simulink model "vehicle_body_v2"  (R2020b)
settings: Solver=VariableStepAuto  StartTime=0.0  StopTime=10.0  RelTol=1e-3
libraries: sdl_lib x14, nesl_utility x8, autolibshared x1
settings Model: Creator=True  LastModifiedBy=True

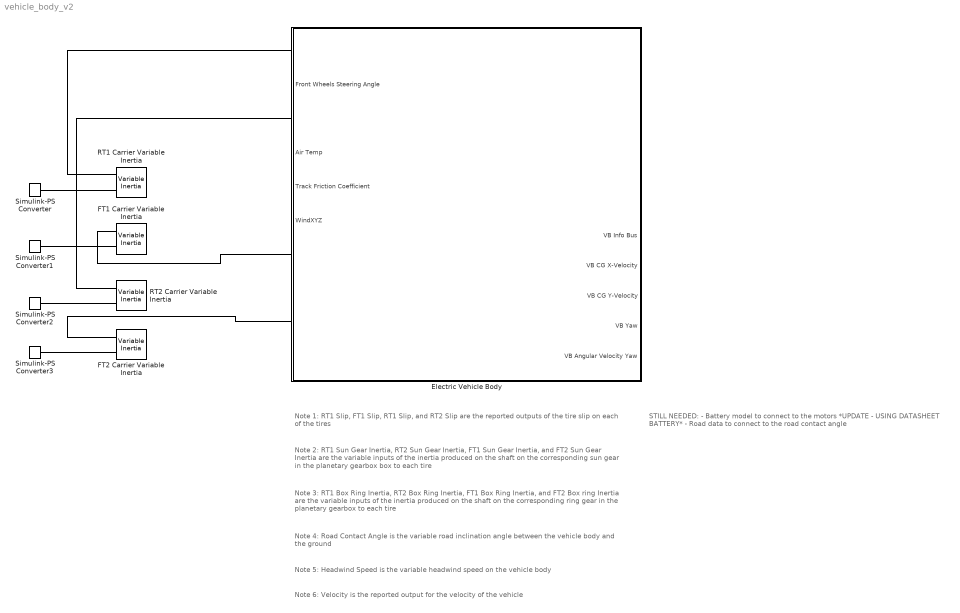
== system vehicle_body_v2 ==
  note: STILL NEEDED:
      |
      | - Battery model to connect to the motors *UPDATE - USING DATASHEET BATTERY*
      |
      | - Road data to connect to the road contact angle
  note: Note 6: Velocity is the reported output for the velocity of the vehicle
  note: Note 5: Headwind Speed is the variable headwind speed on the vehicle body
  note: Note 4: Road Contact Angle is the variable road inclination angle between the vehicle body and the ground
  note: Note 3: RT1 Box Ring Inertia, RT2 Box Ring Inertia, FT1 Box Ring Inertia, and FT2 Box ring Inertia are the variable inputs of the inertia produced on the shaft on the corresponding ring gear in the planetary gearbox to each tire
  note: Note 2: RT1 Sun Gear Inertia, RT2 Sun Gear Inertia, FT1 Sun Gear Inertia, and FT2 Sun Gear Inertia are the variable inputs of the inertia produced on the shaft on the corresponding sun gear in the planetary gearbox box to each tire
  note: Note 1: RT1 Slip, FT1 Slip, RT1 Slip, and RT2 Slip are the reported outputs of the tire slip on each of the tires
  Electric Vehicle Body : Subsystem
      settings: PortSchema="{\"entries\":[{\"content\":{\"sides\":[{\"content\":{\"connectorIds\":[\"LConn1\",\"In1\",\"LConn2\",\"In2\",\"In3\",\"In4\",\"LConn3\",\"LConn4\",\"LConn5\",\"LConn6\"]},\"type\":\"ConnectorPlacement.EquallySpacedRectSide\",\"uuid\":\"3589ffd8-3282-449f-9f73-db5573b89272\"},{\"content\":{\"connectorIds\":[\"RConn1\",\"RConn2\",\"RConn3\",\"RConn4\",\"RConn5\",\"RConn6\",\"Out1\",\"Out2\",\"Out3\",\"Out4\",\"Out5\"],\"side\":\"RIGHT\"},\"type\":\"ConnectorPlacement.EquallySpacedRectSide\",\"uuid\":\"4bc75fc4-5a6d-4cdc-a1d8-7589f1bfd0e3\"},{\"content\":{\"connectorIds\":[],\"side\":\"TOP\"},\"type\":\"ConnectorPlacement.EquallySpacedRectSide\",\"uuid\":\"5582f31c-489d-4354-9c03-0beb1d144974\"},{\"content\":{\"connectorIds\":[],\"side\":\"HIDDEN\"},\"type\":\"ConnectorPlacement.EquallySpacedRectSide\",\"uuid\":\"95051cab-6025-4def-8e94-855365c64cfc\"}]},\"type\":\"ConnectorPlacement.EquallySpacedConnector\",\"uuid\":\"f0af1aeb-7bbe-491f-85c8-fb0f3026e409\"}],\"packageUris\":[\"http://schema.mathworks.com/mf0/Connector/R2020b\"],\"version\":\"1.0\"}"
  FT1 Carrier Variable Inertia : sdl_lib/Inertias & Loads/Variable Inertia  minimum_inertia=0.1 kg*m^2  L_specify=off  L_priority=High  L=0 m^2*kg/s  L_nominal_specify=off  L_nominal_unit=m^2*kg/s  L_nominal_value=1
      settings: SourceProductBaseCode=LD  InternalSimscapePortConfiguration="{\"Bottom\":[],\"Left\":[{\"id\":\"I\",\"label\":\"\",\"type\":\"input\"},{\"id\":\"A\",\"label\":\"\",\"type\":\"foundation.mechanical.rotational.rotational\"}],\"Right\":[],\"Top\":[]}"
  FT2 Carrier Variable Inertia : sdl_lib/Inertias & Loads/Variable Inertia  minimum_inertia=0.1 kg*m^2  L_specify=off  L_priority=High  L=0 m^2*kg/s  L_nominal_specify=off  L_nominal_unit=m^2*kg/s  L_nominal_value=1
      settings: SourceProductBaseCode=LD  InternalSimscapePortConfiguration="{\"Bottom\":[],\"Left\":[{\"id\":\"I\",\"label\":\"\",\"type\":\"input\"},{\"id\":\"A\",\"label\":\"\",\"type\":\"foundation.mechanical.rotational.rotational\"}],\"Right\":[],\"Top\":[]}"
  RT1 Carrier Variable Inertia : sdl_lib/Inertias & Loads/Variable Inertia  minimum_inertia=0.1 kg*m^2  L_specify=off  L_priority=High  L=0 m^2*kg/s  L_nominal_specify=off  L_nominal_unit=m^2*kg/s  L_nominal_value=1
      settings: SourceProductBaseCode=LD  InternalSimscapePortConfiguration="{\"Bottom\":[],\"Left\":[{\"id\":\"I\",\"label\":\"\",\"type\":\"input\"},{\"id\":\"A\",\"label\":\"\",\"type\":\"foundation.mechanical.rotational.rotational\"}],\"Right\":[],\"Top\":[]}"
  RT2 Carrier Variable Inertia : sdl_lib/Inertias & Loads/Variable Inertia  minimum_inertia=0.1 kg*m^2  L_specify=off  L_priority=High  L=0 m^2*kg/s  L_nominal_specify=off  L_nominal_unit=m^2*kg/s  L_nominal_value=1
      settings: SourceProductBaseCode=LD  InternalSimscapePortConfiguration="{\"Bottom\":[],\"Left\":[{\"id\":\"I\",\"label\":\"\",\"type\":\"input\"},{\"id\":\"A\",\"label\":\"\",\"type\":\"foundation.mechanical.rotational.rotational\"}],\"Right\":[],\"Top\":[]}"
  Simulink-PS Converter{,1..3} (4 alike) : nesl_utility/Simulink-PS Converter  PhysicalDomain=network_engine_domain  SubClassName=ps_input  LeftPortType=input  RightPortType=output  PseudoPeriodic=off  Frequencies=[]  NoiseDistribution=none  NoiseParameters=[]  Unit=1  AffineConversion=off  FilteringAndDerivatives=provide  SimscapeFilterOrder=1  InputFilterTimeConstant=0.001  UdotUserProvided=0
  connections:
  Simulink-PS Converter1/RConn1 -- FT1 Carrier Variable Inertia/LConn1
  Simulink-PS Converter3/RConn1 -- FT2 Carrier Variable Inertia/LConn1
  FT1 Carrier Variable Inertia/LConn2 -- Electric Vehicle Body/LConn3
  RT2 Carrier Variable Inertia/LConn2 -- Electric Vehicle Body/LConn2
  Simulink-PS Converter/RConn1 -- RT1 Carrier Variable Inertia/LConn1
  FT2 Carrier Variable Inertia/LConn2 -- Electric Vehicle Body/LConn5
  RT1 Carrier Variable Inertia/LConn2 -- Electric Vehicle Body/LConn1
  Simulink-PS Converter2/RConn1 -- RT2 Carrier Variable Inertia/LConn1

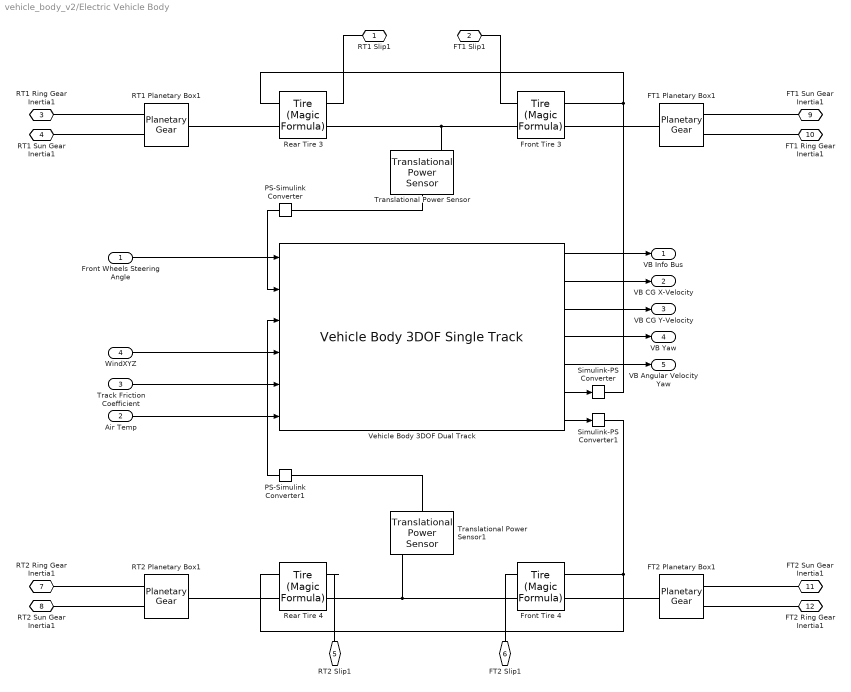
== system vehicle_body_v2/Electric Vehicle Body ==
  Front Wheels Steering Angle : Inport
  Air Temp : Inport  Port=2
  Track Friction Coefficient : Inport  Port=3
  WindXYZ : Inport  Port=4
  FT1 Planetary Box1 : sdl_lib/Gears/Planetary Gear  rs_ratio=2  friction_model=sdl.enum.gear_friction.none  mu_visc=[0, 0] N*m/(rad/s)  efficiency=[.96, .98]  temperature_TLU=[280, 300, 320] K  efficiency_sp_TLU=[.95, .9, .85]  efficiency_rp_TLU=[.95, .9, .85]  pwr_thr=[.001, .001] W  thermal_mass=50 J/K  T_init=300 K  model_inertia=simscape.enum.onoff.off  planet_inertia=0.001 kg*m^2
      settings: SourceProductBaseCode=LD
  FT2 Planetary Box1 : sdl_lib/Gears/Planetary Gear  rs_ratio=2  friction_model=sdl.enum.gear_friction.none  mu_visc=[0, 0] N*m/(rad/s)  efficiency=[.96, .98]  temperature_TLU=[280, 300, 320] K  efficiency_sp_TLU=[.95, .9, .85]  efficiency_rp_TLU=[.95, .9, .85]  pwr_thr=[.001, .001] W  thermal_mass=50 J/K  T_init=300 K  model_inertia=simscape.enum.onoff.off  planet_inertia=0.001 kg*m^2
      settings: SourceProductBaseCode=LD
  Front Tire 3 : sdl_lib/Tires & Vehicles/Tire (Magic Formula)  parameterization=sdl.enum.magic_tire_model.peak  F_z1=3000 N  F_x1=3500 N  kappa1=10  B_m=10  C_m=1.9  D_m=1  E_m=0.97  fz0=4000 N  p_Cx=1.685  p_Dx=[1.21, -.037]  p_Ex=[.344, .095, -.02, 0]  p_Kx=[21.51, -.163, .245]  p_Hx=[-.002, .002]  p_Vx=[0, 0]  v_tr_thr=0.1 m/s  r_e=0.3 m  model_compliance=0  stiffness=1e6 N/m  damping=1000 N/(m/s)  model_inertia=0  inertia=1 kg*m^2  initial_velocity=0 rad/s  model_resistance=0  resistance_model=1  coeff=0.015  p_tire=250e3 Pa  alpha=-0.003  beta=0.97  coeff_a=84e-4  coeff_b=6.2e-4 s/m  coeff_c=1.6e-4 s^2/m^2  v_thr=0.001 m/s
  Front Tire 4 : sdl_lib/Tires & Vehicles/Tire (Magic Formula)  parameterization=sdl.enum.magic_tire_model.peak  F_z1=3000 N  F_x1=3500 N  kappa1=10  B_m=10  C_m=1.9  D_m=1  E_m=0.97  fz0=4000 N  p_Cx=1.685  p_Dx=[1.21, -.037]  p_Ex=[.344, .095, -.02, 0]  p_Kx=[21.51, -.163, .245]  p_Hx=[-.002, .002]  p_Vx=[0, 0]  v_tr_thr=0.1 m/s  r_e=0.3 m  model_compliance=0  stiffness=1e6 N/m  damping=1000 N/(m/s)  model_inertia=0  inertia=1 kg*m^2  initial_velocity=0 rad/s  model_resistance=0  resistance_model=1  coeff=0.015  p_tire=250e3 Pa  alpha=-0.003  beta=0.97  coeff_a=84e-4  coeff_b=6.2e-4 s/m  coeff_c=1.6e-4 s^2/m^2  v_thr=0.001 m/s
  PS-Simulink Converter : nesl_utility/PS-Simulink Converter  PhysicalDomain=network_engine_domain  SubClassName=ps_output  LeftPortType=input  RightPortType=output  PseudoPeriodic=off  Frequencies=[]  Unit=inherit  AffineConversion=off
  PS-Simulink Converter1 : nesl_utility/PS-Simulink Converter  PhysicalDomain=network_engine_domain  SubClassName=ps_output  LeftPortType=input  RightPortType=output  PseudoPeriodic=off  Frequencies=[]  Unit=inherit  AffineConversion=off
  RT1 Planetary Box1 : sdl_lib/Gears/Planetary Gear  rs_ratio=2  friction_model=sdl.enum.gear_friction.none  mu_visc=[0, 0] N*m/(rad/s)  efficiency=[.96, .98]  temperature_TLU=[280, 300, 320] K  efficiency_sp_TLU=[.95, .9, .85]  efficiency_rp_TLU=[.95, .9, .85]  pwr_thr=[.001, .001] W  thermal_mass=50 J/K  T_init=300 K  model_inertia=simscape.enum.onoff.off  planet_inertia=0.001 kg*m^2
      settings: SourceProductBaseCode=LD
  RT2 Planetary Box1 : sdl_lib/Gears/Planetary Gear  rs_ratio=2  friction_model=sdl.enum.gear_friction.none  mu_visc=[0, 0] N*m/(rad/s)  efficiency=[.96, .98]  temperature_TLU=[280, 300, 320] K  efficiency_sp_TLU=[.95, .9, .85]  efficiency_rp_TLU=[.95, .9, .85]  pwr_thr=[.001, .001] W  thermal_mass=50 J/K  T_init=300 K  model_inertia=simscape.enum.onoff.off  planet_inertia=0.001 kg*m^2
      settings: SourceProductBaseCode=LD
  Rear Tire 3 : sdl_lib/Tires & Vehicles/Tire (Magic Formula)  parameterization=sdl.enum.magic_tire_model.peak  F_z1=3000 N  F_x1=3500 N  kappa1=10  B_m=10  C_m=1.9  D_m=1  E_m=0.97  fz0=4000 N  p_Cx=1.685  p_Dx=[1.21, -.037]  p_Ex=[.344, .095, -.02, 0]  p_Kx=[21.51, -.163, .245]  p_Hx=[-.002, .002]  p_Vx=[0, 0]  v_tr_thr=0.1 m/s  r_e=0.3 m  model_compliance=0  stiffness=1e6 N/m  damping=1000 N/(m/s)  model_inertia=0  inertia=1 kg*m^2  initial_velocity=0 rad/s  model_resistance=0  resistance_model=1  coeff=0.015  p_tire=250e3 Pa  alpha=-0.003  beta=0.97  coeff_a=84e-4  coeff_b=6.2e-4 s/m  coeff_c=1.6e-4 s^2/m^2  v_thr=0.001 m/s
  Rear Tire 4 : sdl_lib/Tires & Vehicles/Tire (Magic Formula)  parameterization=sdl.enum.magic_tire_model.peak  F_z1=3000 N  F_x1=3500 N  kappa1=10  B_m=10  C_m=1.9  D_m=1  E_m=0.97  fz0=4000 N  p_Cx=1.685  p_Dx=[1.21, -.037]  p_Ex=[.344, .095, -.02, 0]  p_Kx=[21.51, -.163, .245]  p_Hx=[-.002, .002]  p_Vx=[0, 0]  v_tr_thr=0.1 m/s  r_e=0.3 m  model_compliance=0  stiffness=1e6 N/m  damping=1000 N/(m/s)  model_inertia=0  inertia=1 kg*m^2  initial_velocity=0 rad/s  model_resistance=0  resistance_model=1  coeff=0.015  p_tire=250e3 Pa  alpha=-0.003  beta=0.97  coeff_a=84e-4  coeff_b=6.2e-4 s/m  coeff_c=1.6e-4 s^2/m^2  v_thr=0.001 m/s
  Simulink-PS Converter : nesl_utility/Simulink-PS Converter  PhysicalDomain=network_engine_domain  SubClassName=ps_input  LeftPortType=input  RightPortType=output  PseudoPeriodic=off  Frequencies=[]  NoiseDistribution=none  NoiseParameters=[]  Unit=1  AffineConversion=off  FilteringAndDerivatives=provide  SimscapeFilterOrder=1  InputFilterTimeConstant=0.001  UdotUserProvided=0
  Simulink-PS Converter1 : nesl_utility/Simulink-PS Converter  PhysicalDomain=network_engine_domain  SubClassName=ps_input  LeftPortType=input  RightPortType=output  PseudoPeriodic=off  Frequencies=[]  NoiseDistribution=none  NoiseParameters=[]  Unit=1  AffineConversion=off  FilteringAndDerivatives=provide  SimscapeFilterOrder=1  InputFilterTimeConstant=0.001  UdotUserProvided=0
  Translational Power Sensor : sdl_lib/Sensors/Translational Power Sensor  measurement_type=1  averaging_period=1 s  max_frequency=1000 Hz
      settings: SourceProductBaseCode=LD  InternalSimscapePortConfiguration="{\"Bottom\":[],\"Left\":[{\"id\":\"S\",\"label\":\"S\",\"type\":\"foundation.mechanical.translational.translational\"},{\"id\":\"R\",\"label\":\"R\",\"type\":\"foundation.mechanical.translational.translational\"},{\"id\":\"C\",\"label\":\"C\",\"type\":\"foundation.mechanical.translational.translational\"}],\"Right\":[{\"id\":\"P\",\"label\":\"P\",\"type\":\"output\"}],\"Top\":[]}"
  Translational Power Sensor1 : sdl_lib/Sensors/Translational Power Sensor  measurement_type=1  averaging_period=1 s  max_frequency=1000 Hz
      settings: SourceProductBaseCode=LD  InternalSimscapePortConfiguration="{\"Bottom\":[],\"Left\":[{\"id\":\"S\",\"label\":\"S\",\"type\":\"foundation.mechanical.translational.translational\"},{\"id\":\"R\",\"label\":\"R\",\"type\":\"foundation.mechanical.translational.translational\"},{\"id\":\"C\",\"label\":\"C\",\"type\":\"foundation.mechanical.translational.translational\"}],\"Right\":[{\"id\":\"P\",\"label\":\"P\",\"type\":\"output\"}],\"Top\":[]}"
  Vehicle Body 3DOF Dual Track : autolibshared/Vehicle Body 3DOF Single Track  trackMode=Dual  inputMode=External longitudinal forces  frontSteerMode=on  rearSteerMode=off  windMode=on  muMode=on  extFMode=off  extMMode=off  htchFMode=off  htchMMode=off  extXo=off  extpsio=off  extxdoto=off  extro=off  extYo=off  extTamb=on  extydoto=off  aMode=2  NF=2  NR=2  m=2000  a=1.4  b=1.6  h=0.35  dh=1  hh=0.2  X_o=0  xdot_o=0  CalphaMode=off  sigmaMode=on  d=0  hl=0  w=[1.4,1.4]  Cy_f=12e3  Cy_r=11e3  sigma_f=.1  sigma_r=.1  alpha_f_brk=[-.1 .1]  Cy_f_data=[-9e3 9e3]  alpha_r_brk=[-.1 .1]  Cy_r_data=[-9e3 9e3]  Y_o=0  ydot_o=0  Izz=4000  psi_o=0  r_o=0  Af=2  Cd=.3  Cl=.1  Cpm=.1  beta_w=[0:0.01:0.3]  Cs=[0:0.03:0.9]  Cym=[0:0.01:0.3]  Pabs=101325  Tair=273  g=9.81  mu=1  xdot_tol=.01  Fznom=5000  Fxtire_sat=7e4  Fytire_sat=7e4  longOff=0  latOff=0  vertOff=0  wrapAng=off
      settings: SourceProductBaseCode=PW,MT,UV,VE,VP
  RT1 Slip1 : PMIOPort  Side=Right
  FT1 Slip1 : PMIOPort  Port=2  Side=Right
  RT1 Ring Gear Inertia1 : PMIOPort  Port=3  Side=Right
  RT1 Sun Gear Inertia1 : PMIOPort  Port=4  Side=Left
  RT2 Slip1 : PMIOPort  Port=5  Side=Right
  FT2 Slip1 : PMIOPort  Port=6  Side=Right
  RT2 Ring Gear Inertia1 : PMIOPort  Port=7  Side=Right
  RT2 Sun Gear Inertia1 : PMIOPort  Port=8  Side=Left
  FT1 Sun Gear Inertia1 : PMIOPort  Port=9  Side=Left
  FT1 Ring Gear Inertia1 : PMIOPort  Port=10  Side=Left
  FT2 Sun Gear Inertia1 : PMIOPort  Port=11  Side=Left
  FT2 Ring Gear Inertia1 : PMIOPort  Port=12  Side=Left
  VB Info Bus : Outport
  "VB CG X-Velocity " : Outport  Port=2
  VB CG Y-Velocity : Outport  Port=3
  VB Yaw : Outport  Port=4
  VB Angular Velocity Yaw : Outport  Port=5
  wires:
  PS-Simulink Converter/1 -> Vehicle Body 3DOF Dual Track/2
  PS-Simulink Converter1/1 -> Vehicle Body 3DOF Dual Track/3
  Vehicle Body 3DOF Dual Track/6 -> Simulink-PS Converter/1
  Vehicle Body 3DOF Dual Track/7 -> Simulink-PS Converter1/1
  Air Temp/1 -> Vehicle Body 3DOF Dual Track/6
  Front Wheels Steering Angle/1 -> Vehicle Body 3DOF Dual Track/1
  Track Friction Coefficient/1 -> Vehicle Body 3DOF Dual Track/5
  WindXYZ/1 -> Vehicle Body 3DOF Dual Track/4
  Vehicle Body 3DOF Dual Track/1 -> VB Info Bus/1
  Vehicle Body 3DOF Dual Track/2 -> "VB CG X-Velocity "/1
  Vehicle Body 3DOF Dual Track/3 -> VB CG Y-Velocity/1
  Vehicle Body 3DOF Dual Track/4 -> VB Yaw/1
  Vehicle Body 3DOF Dual Track/5 -> VB Angular Velocity Yaw/1
  connections:
  Rear Tire 4/RConn2 -- Translational Power Sensor1/LConn1 -- Front Tire 4/RConn2
  RT1 Ring Gear Inertia1/RConn1 -- RT1 Planetary Box1/RConn1
  FT2 Ring Gear Inertia1/RConn1 -- FT2 Planetary Box1/RConn1
  RT2 Ring Gear Inertia1/RConn1 -- RT2 Planetary Box1/RConn1
  Rear Tire 4/LConn2 -- RT2 Planetary Box1/LConn1
  FT2 Sun Gear Inertia1/RConn1 -- FT2 Planetary Box1/RConn2
  Rear Tire 4/RConn1 -- RT2 Slip1/RConn1
  Front Tire 3/RConn1 -- FT1 Slip1/RConn1
  RT2 Sun Gear Inertia1/RConn1 -- RT2 Planetary Box1/RConn2
  Rear Tire 3/RConn1 -- RT1 Slip1/RConn1
  FT1 Ring Gear Inertia1/RConn1 -- FT1 Planetary Box1/RConn1
  Front Tire 4/RConn1 -- FT2 Slip1/RConn1
  FT1 Planetary Box1/LConn1 -- Front Tire 3/LConn2
  Front Tire 4/LConn2 -- FT2 Planetary Box1/LConn1
  RT1 Sun Gear Inertia1/RConn1 -- RT1 Planetary Box1/RConn2
  RT1 Planetary Box1/LConn1 -- Rear Tire 3/LConn2
  FT1 Sun Gear Inertia1/RConn1 -- FT1 Planetary Box1/RConn2
  PS-Simulink Converter/LConn1 -- Translational Power Sensor/RConn1
  Rear Tire 3/RConn2 -- Front Tire 3/RConn2 -- Translational Power Sensor/LConn1
  PS-Simulink Converter1/LConn1 -- Translational Power Sensor1/RConn1
  Simulink-PS Converter/RConn1 -- Rear Tire 3/LConn1 -- Front Tire 3/LConn1
  Simulink-PS Converter1/RConn1 -- Rear Tire 4/LConn1 -- Front Tire 4/LConn1
